simulink model "PLL_fault_experiment"  (R2025a)
settings: Solver=FixedStepAuto  StartTime=0.0  StopTime=1  FixedStep=Ts  RelTol=1e-3
values from neighbouring files (symbols this model uses):
  C_dc = 2.25    [PLLpara.m]
  Cf1 = 0.01    [PLLpara.m]
  Cf2 = 0.01    [PLLpara.m]
  dt_sag = t_c    [GFMPara.m]    (also in GFMPara_exp.m; PLLpara.m; VFMPara.m; VFMPara_exp.m)
  f_switching = 20e3    (= 20000)    [GFMPara_exp.m]    (also in PLLpara.m = 10000; VFMPara_exp.m)
  Id0 = Id    [PLLpara.m]
  Iq01 = 0    [PLLpara.m]
  Iq02 = (Ug*cos(asin((Xg*Id+Rg*Iq)/Ug))+Id*Rg-Iq*Xg)*Cf2+Iq    [PLLpara.m]
  ki_pll1 = ki    [PLLpara.m]
  kp_pll1 = kp    [PLLpara.m]
  Lc = 1e-9    (= 1e-09)    [GFMPara.m]    (also in GFMPara_exp.m; PLLpara.m; VFMPara.m; VFMPara_exp.m)
  Lf = 0.0592    [GFMPara.m]    (also in GFMPara_exp.m; PLLpara.m = 0.05; VFMPara.m = 0.05; VFMPara_exp.m = 0.05)
  Lg1 = X1    [PLLpara.m]    (also in VFMPara.m; VFMPara_exp.m)
  Lgg = Xgg    [PLLpara.m]    (also in VFMPara.m; VFMPara_exp.m)
  Rf = 1e-3    (= 0.001)    [PLLpara.m]
  Rg1 = R1    [PLLpara.m]    (also in VFMPara.m; VFMPara_exp.m = 4*R1/5)
  Rgg = Rgg    [PLLpara.m]    (also in VFMPara.m; VFMPara_exp.m)
  Sbase = 1    [GFMPara.m]    (also in GFMPara_exp.m; PLLpara.m; VFMPara.m; VFMPara_exp.m)
  t0 = t_sim_start +t_start    [PLLpara.m]    (also in VFMPara_exp.m)
  t0_sag = t_sim_start +t_start    [GFMPara.m]    (also in GFMPara_exp.m; PLLpara.m = 20; VFMPara.m; VFMPara_exp.m = 20)
  Tc = 1/f_switching    (= 5e-05)    [GFMPara_exp.m]    (also in PLLpara.m = 0.0001; VFMPara_exp.m)
  tc = t_c    [PLLpara.m]    (also in VFMPara_exp.m)
  Ts = 1/Fs    (= 1e-05)    [GFMPara.m]    (also in GFMPara_exp.m = 1e-06; PLLpara.m = 1e-06; VFMPara.m = 5e-06; VFMPara_exp.m = 1e-06)
  v_sag = Ug_fault    [GFMPara.m]    (also in GFMPara_exp.m; PLLpara.m; VFMPara.m; VFMPara_exp.m)
  Vbase = 1    [GFMPara.m]    (also in GFMPara_exp.m; PLLpara.m; VFMPara.m; VFMPara_exp.m)
  Vdc = 2.5    [PLLpara.m]
  w_i_GFL1 = 1100 *2*pi    (= 6911.5038379)    [PLLpara.m]
  w_i_GFL2 = 1100 *2*pi    (= 6911.5038379)    [PLLpara.m]
  w_pll1 = 10 *2*pi    (= 62.8318530718)    [PLLpara.m]
  w_tau1 = 1500 *2*pi    (= 9424.77796077)    [PLLpara.m]
  Wbase = 2*pi*50    (= 314.159265359)    [GFMPara.m]    (also in GFMPara_exp.m; PLLpara.m; VFMPara.m; VFMPara_exp.m)
  Zbase = Vbase/Ibase    (= 1)    [GFMPara.m]    (also in GFMPara_exp.m; PLLpara.m; VFMPara.m; VFMPara_exp.m)
undefined symbols (not defined in the file or in its folder): DiscIntNeverNeededParam, initial, position, postfault_SEP, sigbuilder_block, w_max, w_min, Ws
libraries: spsVoltageMeasurementLib x80, spsCurrentMeasurementLib x75, spsIdealSwitchLib x30, spsThreePhaseSeriesRLCBranchLib x21, spsControlledVoltageSourceLib x18, spsSeriesRLCBranchLib x11, powerlib_extras x10, spsHalfBridgeConverterLib x6, spsThreePhaseBreakerLib x6, spsDCVoltageSourceLib x4, spsThreePhaseFaultLib x3, cstblocks x2
(part 3 of 5)

== system PLL_fault_experiment/measurement12 ==
  Mux1 : Mux  Inputs=3
  Mux2 : Mux  Inputs=3
  ila : spsCurrentMeasurementLib/Current Measurement  PhasorSimulation=off  OutputType=Complex  PSBequivalent=0
  ilb : spsCurrentMeasurementLib/Current Measurement  PhasorSimulation=off  OutputType=Complex  PSBequivalent=0
  ilc : spsCurrentMeasurementLib/Current Measurement  PhasorSimulation=off  OutputType=Complex  PSBequivalent=0
  vca measure : spsVoltageMeasurementLib/Voltage Measurement  PhasorSimulation=off  OutputType=Complex  PSBequivalent=0
  vcb measure : spsVoltageMeasurementLib/Voltage Measurement  PhasorSimulation=off  OutputType=Complex  PSBequivalent=0
  vcc measure : spsVoltageMeasurementLib/Voltage Measurement  PhasorSimulation=off  OutputType=Complex  PSBequivalent=0
  a : PMIOPort  Side=Left
  b : PMIOPort  Port=2  Side=Left
  c : PMIOPort  Port=3  Side=Left
  n : PMIOPort  Port=4  Side=Left
  A : PMIOPort  Port=5  Side=Right
  B : PMIOPort  Port=6  Side=Right
  C : PMIOPort  Port=7  Side=Right
  N : PMIOPort  Port=8  Side=Right
  Iabc : Outport
  Vabc : Outport  Port=2
  wires:
  ila/1 -> Mux2/1
  ilb/1 -> Mux2/2
  ilc/1 -> Mux2/3
  Mux2/1 -> Iabc/1
  vcb measure/1 -> Mux1/2
  vca measure/1 -> Mux1/1
  vcc measure/1 -> Mux1/3
  Mux1/1 -> Vabc/1
  connections:
  a/RConn1 -- ila/LConn1
  ila/RConn1 -- A/RConn1 -- vca measure/LConn1
  ilb/LConn1 -- b/RConn1
  ilb/RConn1 -- B/RConn1 -- vcb measure/LConn1
  c/RConn1 -- ilc/LConn1
  C/RConn1 -- ilc/RConn1 -- vcc measure/LConn1
  n/RConn1 -- vcc measure/LConn2 -- vcb measure/LConn2 -- vca measure/LConn2 -- N/RConn1

== system PLL_fault_experiment/measurement13 ==
  Mux1 : Mux  Inputs=3
  Mux2 : Mux  Inputs=3
  ila : spsCurrentMeasurementLib/Current Measurement  PhasorSimulation=off  OutputType=Complex  PSBequivalent=0
  ilb : spsCurrentMeasurementLib/Current Measurement  PhasorSimulation=off  OutputType=Complex  PSBequivalent=0
  ilc : spsCurrentMeasurementLib/Current Measurement  PhasorSimulation=off  OutputType=Complex  PSBequivalent=0
  vca measure : spsVoltageMeasurementLib/Voltage Measurement  PhasorSimulation=off  OutputType=Complex  PSBequivalent=0
  vcb measure : spsVoltageMeasurementLib/Voltage Measurement  PhasorSimulation=off  OutputType=Complex  PSBequivalent=0
  vcc measure : spsVoltageMeasurementLib/Voltage Measurement  PhasorSimulation=off  OutputType=Complex  PSBequivalent=0
  a : PMIOPort  Side=Left
  b : PMIOPort  Port=2  Side=Left
  c : PMIOPort  Port=3  Side=Left
  n : PMIOPort  Port=4  Side=Left
  A : PMIOPort  Port=5  Side=Right
  B : PMIOPort  Port=6  Side=Right
  C : PMIOPort  Port=7  Side=Right
  N : PMIOPort  Port=8  Side=Right
  Iabc : Outport
  Vabc : Outport  Port=2
  wires:
  ila/1 -> Mux2/1
  ilb/1 -> Mux2/2
  ilc/1 -> Mux2/3
  Mux2/1 -> Iabc/1
  vcb measure/1 -> Mux1/2
  vca measure/1 -> Mux1/1
  vcc measure/1 -> Mux1/3
  Mux1/1 -> Vabc/1
  connections:
  a/RConn1 -- ila/LConn1
  ila/RConn1 -- A/RConn1 -- vca measure/LConn1
  ilb/LConn1 -- b/RConn1
  ilb/RConn1 -- B/RConn1 -- vcb measure/LConn1
  c/RConn1 -- ilc/LConn1
  C/RConn1 -- ilc/RConn1 -- vcc measure/LConn1
  n/RConn1 -- vcc measure/LConn2 -- vcb measure/LConn2 -- vca measure/LConn2 -- N/RConn1

== system PLL_fault_experiment/measurement14 ==
  Mux1 : Mux  Inputs=3
  Mux2 : Mux  Inputs=3
  ila : spsCurrentMeasurementLib/Current Measurement  PhasorSimulation=off  OutputType=Complex  PSBequivalent=0
  ilb : spsCurrentMeasurementLib/Current Measurement  PhasorSimulation=off  OutputType=Complex  PSBequivalent=0
  ilc : spsCurrentMeasurementLib/Current Measurement  PhasorSimulation=off  OutputType=Complex  PSBequivalent=0
  vca measure : spsVoltageMeasurementLib/Voltage Measurement  PhasorSimulation=off  OutputType=Complex  PSBequivalent=0
  vcb measure : spsVoltageMeasurementLib/Voltage Measurement  PhasorSimulation=off  OutputType=Complex  PSBequivalent=0
  vcc measure : spsVoltageMeasurementLib/Voltage Measurement  PhasorSimulation=off  OutputType=Complex  PSBequivalent=0
  a : PMIOPort  Side=Left
  b : PMIOPort  Port=2  Side=Left
  c : PMIOPort  Port=3  Side=Left
  n : PMIOPort  Port=4  Side=Left
  A : PMIOPort  Port=5  Side=Right
  B : PMIOPort  Port=6  Side=Right
  C : PMIOPort  Port=7  Side=Right
  N : PMIOPort  Port=8  Side=Right
  Iabc : Outport
  Vabc : Outport  Port=2
  wires:
  ila/1 -> Mux2/1
  ilb/1 -> Mux2/2
  ilc/1 -> Mux2/3
  Mux2/1 -> Iabc/1
  vcb measure/1 -> Mux1/2
  vca measure/1 -> Mux1/1
  vcc measure/1 -> Mux1/3
  Mux1/1 -> Vabc/1
  connections:
  a/RConn1 -- ila/LConn1
  ila/RConn1 -- A/RConn1 -- vca measure/LConn1
  ilb/LConn1 -- b/RConn1
  ilb/RConn1 -- B/RConn1 -- vcb measure/LConn1
  c/RConn1 -- ilc/LConn1
  C/RConn1 -- ilc/RConn1 -- vcc measure/LConn1
  n/RConn1 -- vcc measure/LConn2 -- vcb measure/LConn2 -- vca measure/LConn2 -- N/RConn1

== system PLL_fault_experiment/measurement15 ==
  Mux1 : Mux  Inputs=3
  Mux2 : Mux  Inputs=3
  ila : spsCurrentMeasurementLib/Current Measurement  PhasorSimulation=off  OutputType=Complex  PSBequivalent=0
  ilb : spsCurrentMeasurementLib/Current Measurement  PhasorSimulation=off  OutputType=Complex  PSBequivalent=0
  ilc : spsCurrentMeasurementLib/Current Measurement  PhasorSimulation=off  OutputType=Complex  PSBequivalent=0
  vca measure : spsVoltageMeasurementLib/Voltage Measurement  PhasorSimulation=off  OutputType=Complex  PSBequivalent=0
  vcb measure : spsVoltageMeasurementLib/Voltage Measurement  PhasorSimulation=off  OutputType=Complex  PSBequivalent=0
  vcc measure : spsVoltageMeasurementLib/Voltage Measurement  PhasorSimulation=off  OutputType=Complex  PSBequivalent=0
  a : PMIOPort  Side=Left
  b : PMIOPort  Port=2  Side=Left
  c : PMIOPort  Port=3  Side=Left
  n : PMIOPort  Port=4  Side=Left
  A : PMIOPort  Port=5  Side=Right
  B : PMIOPort  Port=6  Side=Right
  C : PMIOPort  Port=7  Side=Right
  N : PMIOPort  Port=8  Side=Right
  Iabc : Outport
  Vabc : Outport  Port=2
  wires:
  ila/1 -> Mux2/1
  ilb/1 -> Mux2/2
  ilc/1 -> Mux2/3
  Mux2/1 -> Iabc/1
  vcb measure/1 -> Mux1/2
  vca measure/1 -> Mux1/1
  vcc measure/1 -> Mux1/3
  Mux1/1 -> Vabc/1
  connections:
  a/RConn1 -- ila/LConn1
  ila/RConn1 -- A/RConn1 -- vca measure/LConn1
  ilb/LConn1 -- b/RConn1
  ilb/RConn1 -- B/RConn1 -- vcb measure/LConn1
  c/RConn1 -- ilc/LConn1
  C/RConn1 -- ilc/RConn1 -- vcc measure/LConn1
  n/RConn1 -- vcc measure/LConn2 -- vcb measure/LConn2 -- vca measure/LConn2 -- N/RConn1

== system PLL_fault_experiment/measurement2 ==
  Mux1 : Mux  Inputs=3
  Mux2 : Mux  Inputs=3
  ila : spsCurrentMeasurementLib/Current Measurement  PhasorSimulation=off  OutputType=Complex  PSBequivalent=0
  ilb : spsCurrentMeasurementLib/Current Measurement  PhasorSimulation=off  OutputType=Complex  PSBequivalent=0
  ilc : spsCurrentMeasurementLib/Current Measurement  PhasorSimulation=off  OutputType=Complex  PSBequivalent=0
  vca measure : spsVoltageMeasurementLib/Voltage Measurement  PhasorSimulation=off  OutputType=Complex  PSBequivalent=0
  vcb measure : spsVoltageMeasurementLib/Voltage Measurement  PhasorSimulation=off  OutputType=Complex  PSBequivalent=0
  vcc measure : spsVoltageMeasurementLib/Voltage Measurement  PhasorSimulation=off  OutputType=Complex  PSBequivalent=0
  a : PMIOPort  Side=Left
  b : PMIOPort  Port=2  Side=Left
  c : PMIOPort  Port=3  Side=Left
  n : PMIOPort  Port=4  Side=Left
  A : PMIOPort  Port=5  Side=Right
  B : PMIOPort  Port=6  Side=Right
  C : PMIOPort  Port=7  Side=Right
  N : PMIOPort  Port=8  Side=Right
  Iabc : Outport
  Vabc : Outport  Port=2
  wires:
  ila/1 -> Mux2/1
  ilb/1 -> Mux2/2
  ilc/1 -> Mux2/3
  Mux2/1 -> Iabc/1
  vcb measure/1 -> Mux1/2
  vca measure/1 -> Mux1/1
  vcc measure/1 -> Mux1/3
  Mux1/1 -> Vabc/1
  connections:
  a/RConn1 -- ila/LConn1
  ila/RConn1 -- A/RConn1 -- vca measure/LConn1
  ilb/LConn1 -- b/RConn1
  ilb/RConn1 -- B/RConn1 -- vcb measure/LConn1
  c/RConn1 -- ilc/LConn1
  C/RConn1 -- ilc/RConn1 -- vcc measure/LConn1
  n/RConn1 -- vcc measure/LConn2 -- vcb measure/LConn2 -- vca measure/LConn2 -- N/RConn1

== system PLL_fault_experiment/measurement3 ==
  Mux1 : Mux  Inputs=3
  Mux2 : Mux  Inputs=3
  ila : spsCurrentMeasurementLib/Current Measurement  PhasorSimulation=off  OutputType=Complex  PSBequivalent=0
  ilb : spsCurrentMeasurementLib/Current Measurement  PhasorSimulation=off  OutputType=Complex  PSBequivalent=0
  ilc : spsCurrentMeasurementLib/Current Measurement  PhasorSimulation=off  OutputType=Complex  PSBequivalent=0
  vca measure : spsVoltageMeasurementLib/Voltage Measurement  PhasorSimulation=off  OutputType=Complex  PSBequivalent=0
  vcb measure : spsVoltageMeasurementLib/Voltage Measurement  PhasorSimulation=off  OutputType=Complex  PSBequivalent=0
  vcc measure : spsVoltageMeasurementLib/Voltage Measurement  PhasorSimulation=off  OutputType=Complex  PSBequivalent=0
  a : PMIOPort  Side=Left
  b : PMIOPort  Port=2  Side=Left
  c : PMIOPort  Port=3  Side=Left
  n : PMIOPort  Port=4  Side=Left
  A : PMIOPort  Port=5  Side=Right
  B : PMIOPort  Port=6  Side=Right
  C : PMIOPort  Port=7  Side=Right
  N : PMIOPort  Port=8  Side=Right
  Iabc : Outport
  Vabc : Outport  Port=2
  wires:
  ila/1 -> Mux2/1
  ilb/1 -> Mux2/2
  ilc/1 -> Mux2/3
  Mux2/1 -> Iabc/1
  vcb measure/1 -> Mux1/2
  vca measure/1 -> Mux1/1
  vcc measure/1 -> Mux1/3
  Mux1/1 -> Vabc/1
  connections:
  a/RConn1 -- ila/LConn1
  ila/RConn1 -- A/RConn1 -- vca measure/LConn1
  ilb/LConn1 -- b/RConn1
  ilb/RConn1 -- B/RConn1 -- vcb measure/LConn1
  c/RConn1 -- ilc/LConn1
  C/RConn1 -- ilc/RConn1 -- vcc measure/LConn1
  n/RConn1 -- vcc measure/LConn2 -- vcb measure/LConn2 -- vca measure/LConn2 -- N/RConn1

== system PLL_fault_experiment/measurement4 ==
  Mux1 : Mux  Inputs=3
  Mux2 : Mux  Inputs=3
  ila : spsCurrentMeasurementLib/Current Measurement  PhasorSimulation=off  OutputType=Complex  PSBequivalent=0
  ilb : spsCurrentMeasurementLib/Current Measurement  PhasorSimulation=off  OutputType=Complex  PSBequivalent=0
  ilc : spsCurrentMeasurementLib/Current Measurement  PhasorSimulation=off  OutputType=Complex  PSBequivalent=0
  vca measure : spsVoltageMeasurementLib/Voltage Measurement  PhasorSimulation=off  OutputType=Complex  PSBequivalent=0
  vcb measure : spsVoltageMeasurementLib/Voltage Measurement  PhasorSimulation=off  OutputType=Complex  PSBequivalent=0
  vcc measure : spsVoltageMeasurementLib/Voltage Measurement  PhasorSimulation=off  OutputType=Complex  PSBequivalent=0
  a : PMIOPort  Side=Left
  b : PMIOPort  Port=2  Side=Left
  c : PMIOPort  Port=3  Side=Left
  n : PMIOPort  Port=4  Side=Left
  A : PMIOPort  Port=5  Side=Right
  B : PMIOPort  Port=6  Side=Right
  C : PMIOPort  Port=7  Side=Right
  N : PMIOPort  Port=8  Side=Right
  Iabc : Outport
  Vabc : Outport  Port=2
  wires:
  ila/1 -> Mux2/1
  ilb/1 -> Mux2/2
  ilc/1 -> Mux2/3
  Mux2/1 -> Iabc/1
  vcb measure/1 -> Mux1/2
  vca measure/1 -> Mux1/1
  vcc measure/1 -> Mux1/3
  Mux1/1 -> Vabc/1
  connections:
  a/RConn1 -- ila/LConn1
  ila/RConn1 -- A/RConn1 -- vca measure/LConn1
  ilb/LConn1 -- b/RConn1
  ilb/RConn1 -- B/RConn1 -- vcb measure/LConn1
  c/RConn1 -- ilc/LConn1
  C/RConn1 -- ilc/RConn1 -- vcc measure/LConn1
  n/RConn1 -- vcc measure/LConn2 -- vcb measure/LConn2 -- vca measure/LConn2 -- N/RConn1

== system PLL_fault_experiment/measurement5 ==
  Mux1 : Mux  Inputs=3
  Mux2 : Mux  Inputs=3
  ila : spsCurrentMeasurementLib/Current Measurement  PhasorSimulation=off  OutputType=Complex  PSBequivalent=0
  ilb : spsCurrentMeasurementLib/Current Measurement  PhasorSimulation=off  OutputType=Complex  PSBequivalent=0
  ilc : spsCurrentMeasurementLib/Current Measurement  PhasorSimulation=off  OutputType=Complex  PSBequivalent=0
  vca measure : spsVoltageMeasurementLib/Voltage Measurement  PhasorSimulation=off  OutputType=Complex  PSBequivalent=0
  vcb measure : spsVoltageMeasurementLib/Voltage Measurement  PhasorSimulation=off  OutputType=Complex  PSBequivalent=0
  vcc measure : spsVoltageMeasurementLib/Voltage Measurement  PhasorSimulation=off  OutputType=Complex  PSBequivalent=0
  a : PMIOPort  Side=Left
  b : PMIOPort  Port=2  Side=Left
  c : PMIOPort  Port=3  Side=Left
  n : PMIOPort  Port=4  Side=Left
  A : PMIOPort  Port=5  Side=Right
  B : PMIOPort  Port=6  Side=Right
  C : PMIOPort  Port=7  Side=Right
  N : PMIOPort  Port=8  Side=Right
  Iabc : Outport
  Vabc : Outport  Port=2
  wires:
  ila/1 -> Mux2/1
  ilb/1 -> Mux2/2
  ilc/1 -> Mux2/3
  Mux2/1 -> Iabc/1
  vcb measure/1 -> Mux1/2
  vca measure/1 -> Mux1/1
  vcc measure/1 -> Mux1/3
  Mux1/1 -> Vabc/1
  connections:
  a/RConn1 -- ila/LConn1
  ila/RConn1 -- A/RConn1 -- vca measure/LConn1
  ilb/LConn1 -- b/RConn1
  ilb/RConn1 -- B/RConn1 -- vcb measure/LConn1
  c/RConn1 -- ilc/LConn1
  C/RConn1 -- ilc/RConn1 -- vcc measure/LConn1
  n/RConn1 -- vcc measure/LConn2 -- vcb measure/LConn2 -- vca measure/LConn2 -- N/RConn1

== system PLL_fault_experiment/measurement6 ==
  Mux1 : Mux  Inputs=3
  Mux2 : Mux  Inputs=3
  ila : spsCurrentMeasurementLib/Current Measurement  PhasorSimulation=off  OutputType=Complex  PSBequivalent=0
  ilb : spsCurrentMeasurementLib/Current Measurement  PhasorSimulation=off  OutputType=Complex  PSBequivalent=0
  ilc : spsCurrentMeasurementLib/Current Measurement  PhasorSimulation=off  OutputType=Complex  PSBequivalent=0
  vca measure : spsVoltageMeasurementLib/Voltage Measurement  PhasorSimulation=off  OutputType=Complex  PSBequivalent=0
  vcb measure : spsVoltageMeasurementLib/Voltage Measurement  PhasorSimulation=off  OutputType=Complex  PSBequivalent=0
  vcc measure : spsVoltageMeasurementLib/Voltage Measurement  PhasorSimulation=off  OutputType=Complex  PSBequivalent=0
  a : PMIOPort  Side=Left
  b : PMIOPort  Port=2  Side=Left
  c : PMIOPort  Port=3  Side=Left
  n : PMIOPort  Port=4  Side=Left
  A : PMIOPort  Port=5  Side=Right
  B : PMIOPort  Port=6  Side=Right
  C : PMIOPort  Port=7  Side=Right
  N : PMIOPort  Port=8  Side=Right
  Iabc : Outport
  Vabc : Outport  Port=2
  wires:
  ila/1 -> Mux2/1
  ilb/1 -> Mux2/2
  ilc/1 -> Mux2/3
  Mux2/1 -> Iabc/1
  vcb measure/1 -> Mux1/2
  vca measure/1 -> Mux1/1
  vcc measure/1 -> Mux1/3
  Mux1/1 -> Vabc/1
  connections:
  a/RConn1 -- ila/LConn1
  ila/RConn1 -- A/RConn1 -- vca measure/LConn1
  ilb/LConn1 -- b/RConn1
  ilb/RConn1 -- B/RConn1 -- vcb measure/LConn1
  c/RConn1 -- ilc/LConn1
  C/RConn1 -- ilc/RConn1 -- vcc measure/LConn1
  n/RConn1 -- vcc measure/LConn2 -- vcb measure/LConn2 -- vca measure/LConn2 -- N/RConn1

== system PLL_fault_experiment/measurement7 ==
  Mux1 : Mux  Inputs=3
  Mux2 : Mux  Inputs=3
  ila : spsCurrentMeasurementLib/Current Measurement  PhasorSimulation=off  OutputType=Complex  PSBequivalent=0
  ilb : spsCurrentMeasurementLib/Current Measurement  PhasorSimulation=off  OutputType=Complex  PSBequivalent=0
  ilc : spsCurrentMeasurementLib/Current Measurement  PhasorSimulation=off  OutputType=Complex  PSBequivalent=0
  vca measure : spsVoltageMeasurementLib/Voltage Measurement  PhasorSimulation=off  OutputType=Complex  PSBequivalent=0
  vcb measure : spsVoltageMeasurementLib/Voltage Measurement  PhasorSimulation=off  OutputType=Complex  PSBequivalent=0
  vcc measure : spsVoltageMeasurementLib/Voltage Measurement  PhasorSimulation=off  OutputType=Complex  PSBequivalent=0
  a : PMIOPort  Side=Left
  b : PMIOPort  Port=2  Side=Left
  c : PMIOPort  Port=3  Side=Left
  n : PMIOPort  Port=4  Side=Left
  A : PMIOPort  Port=5  Side=Right
  B : PMIOPort  Port=6  Side=Right
  C : PMIOPort  Port=7  Side=Right
  N : PMIOPort  Port=8  Side=Right
  Iabc : Outport
  Vabc : Outport  Port=2
  wires:
  ila/1 -> Mux2/1
  ilb/1 -> Mux2/2
  ilc/1 -> Mux2/3
  Mux2/1 -> Iabc/1
  vcb measure/1 -> Mux1/2
  vca measure/1 -> Mux1/1
  vcc measure/1 -> Mux1/3
  Mux1/1 -> Vabc/1
  connections:
  a/RConn1 -- ila/LConn1
  ila/RConn1 -- A/RConn1 -- vca measure/LConn1
  ilb/LConn1 -- b/RConn1
  ilb/RConn1 -- B/RConn1 -- vcb measure/LConn1
  c/RConn1 -- ilc/LConn1
  C/RConn1 -- ilc/RConn1 -- vcc measure/LConn1
  n/RConn1 -- vcc measure/LConn2 -- vcb measure/LConn2 -- vca measure/LConn2 -- N/RConn1

== system PLL_fault_experiment/measurement8 ==
  Mux1 : Mux  Inputs=3
  Mux2 : Mux  Inputs=3
  ila : spsCurrentMeasurementLib/Current Measurement  PhasorSimulation=off  OutputType=Complex  PSBequivalent=0
  ilb : spsCurrentMeasurementLib/Current Measurement  PhasorSimulation=off  OutputType=Complex  PSBequivalent=0
  ilc : spsCurrentMeasurementLib/Current Measurement  PhasorSimulation=off  OutputType=Complex  PSBequivalent=0
  vca measure : spsVoltageMeasurementLib/Voltage Measurement  PhasorSimulation=off  OutputType=Complex  PSBequivalent=0
  vcb measure : spsVoltageMeasurementLib/Voltage Measurement  PhasorSimulation=off  OutputType=Complex  PSBequivalent=0
  vcc measure : spsVoltageMeasurementLib/Voltage Measurement  PhasorSimulation=off  OutputType=Complex  PSBequivalent=0
  a : PMIOPort  Side=Left
  b : PMIOPort  Port=2  Side=Left
  c : PMIOPort  Port=3  Side=Left
  n : PMIOPort  Port=4  Side=Left
  A : PMIOPort  Port=5  Side=Right
  B : PMIOPort  Port=6  Side=Right
  C : PMIOPort  Port=7  Side=Right
  N : PMIOPort  Port=8  Side=Right
  Iabc : Outport
  Vabc : Outport  Port=2
  wires:
  ila/1 -> Mux2/1
  ilb/1 -> Mux2/2
  ilc/1 -> Mux2/3
  Mux2/1 -> Iabc/1
  vcb measure/1 -> Mux1/2
  vca measure/1 -> Mux1/1
  vcc measure/1 -> Mux1/3
  Mux1/1 -> Vabc/1
  connections:
  a/RConn1 -- ila/LConn1
  ila/RConn1 -- A/RConn1 -- vca measure/LConn1
  ilb/LConn1 -- b/RConn1
  ilb/RConn1 -- B/RConn1 -- vcb measure/LConn1
  c/RConn1 -- ilc/LConn1
  C/RConn1 -- ilc/RConn1 -- vcc measure/LConn1
  n/RConn1 -- vcc measure/LConn2 -- vcb measure/LConn2 -- vca measure/LConn2 -- N/RConn1

== system PLL_fault_experiment/measurement9 ==
  Mux1 : Mux  Inputs=3
  Mux2 : Mux  Inputs=3
  ila : spsCurrentMeasurementLib/Current Measurement  PhasorSimulation=off  OutputType=Complex  PSBequivalent=0
  ilb : spsCurrentMeasurementLib/Current Measurement  PhasorSimulation=off  OutputType=Complex  PSBequivalent=0
  ilc : spsCurrentMeasurementLib/Current Measurement  PhasorSimulation=off  OutputType=Complex  PSBequivalent=0
  vca measure : spsVoltageMeasurementLib/Voltage Measurement  PhasorSimulation=off  OutputType=Complex  PSBequivalent=0
  vcb measure : spsVoltageMeasurementLib/Voltage Measurement  PhasorSimulation=off  OutputType=Complex  PSBequivalent=0
  vcc measure : spsVoltageMeasurementLib/Voltage Measurement  PhasorSimulation=off  OutputType=Complex  PSBequivalent=0
  a : PMIOPort  Side=Left
  b : PMIOPort  Port=2  Side=Left
  c : PMIOPort  Port=3  Side=Left
  n : PMIOPort  Port=4  Side=Left
  A : PMIOPort  Port=5  Side=Right
  B : PMIOPort  Port=6  Side=Right
  C : PMIOPort  Port=7  Side=Right
  N : PMIOPort  Port=8  Side=Right
  Iabc : Outport
  Vabc : Outport  Port=2
  wires:
  ila/1 -> Mux2/1
  ilb/1 -> Mux2/2
  ilc/1 -> Mux2/3
  Mux2/1 -> Iabc/1
  vcb measure/1 -> Mux1/2
  vca measure/1 -> Mux1/1
  vcc measure/1 -> Mux1/3
  Mux1/1 -> Vabc/1
  connections:
  a/RConn1 -- ila/LConn1
  ila/RConn1 -- A/RConn1 -- vca measure/LConn1
  ilb/LConn1 -- b/RConn1
  ilb/RConn1 -- B/RConn1 -- vcb measure/LConn1
  c/RConn1 -- ilc/LConn1
  C/RConn1 -- ilc/RConn1 -- vcc measure/LConn1
  n/RConn1 -- vcc measure/LConn2 -- vcb measure/LConn2 -- vca measure/LConn2 -- N/RConn1

== system PLL_fault_experiment/AC Infinite Bus (Voltage Type)1/PQ Calculation (dq-Frame)1 ==
  note: Power calculation.
      |
      | Author(s): Yitong Li
      |
      | Notes:
      |
      | The calculation is done in dq frame.
  vdq : Inport
  idq : Inport  Port=2
  Mux : Mux  Inputs=2
  Mux1 : Mux  Inputs=2
  P = vd*id+vq*iq : Fcn  Expr=u[1]*u[3]+u[2]*u[4]
  Q = -vd*iq+vq*id : Fcn  Expr=-u[1]*u[4]+u[2]*u[3]
  pq : Outport
  wires:
  Mux/1 -> pq/1
  P = vd*id+vq*iq/1 -> Mux/1
  vdq/1 -> Mux1/1
  idq/1 -> Mux1/2
  Mux1/1 -> P = vd*id+vq*iq/1, Q = -vd*iq+vq*id/1
  Q = -vd*iq+vq*id/1 -> Mux/2

== system PLL_fault_experiment/AC Infinite Bus (Voltage Type)1/abc -> dq (Power-Invariant)1 ==
  note: Frame transformation from abc to dq.
      |
      | Author(s): Yitong Li
      |
      | Notes:
      |
      | The transformation is power-invariant.
      |
      | theta is the angle that d axis leads a axis.
      |
      | q axis leads d axis by 90 degrees.
  abc : Inport
  theta : Inport  Port=2
  ->d : Fcn  Expr=cos(u(4))*u(1) + cos(u(4)-2/3*pi)*u(2) + cos(u(4)-4/3*pi)*u(3)
  ->q : Fcn  Expr=-sin(u(4))*u(1) - sin(u(4)-2/3*pi)*u(2) - sin(u(4)-4/3*pi)*u(3)
  Gain : Gain  Gain=sqrt(2/3)
  Mux5 : Mux  Inputs=2
  Mux6 : Mux  Inputs=2
  dq : Outport
  wires:
  abc/1 -> Gain/1
  ->d/1 -> Mux6/1
  Gain/1 -> Mux5/1
  theta/1 -> Mux5/2
  ->q/1 -> Mux6/2
  Mux6/1 -> dq/1
  Mux5/1 -> ->d/1, ->q/1

== system PLL_fault_experiment/AC Infinite Bus (Voltage Type)1/dq -> abc (Power-Invariant)1 ==
  note: Frame transformation from dq to abc.
      |
      | Author(s): Yitong Li
      |
      | Notes:
      |
      | The transformation is power-invariant.
      |
      | theta is the angle that dq axis leads alpha/beta axis, specifically, d axis leads alpha axis.
  dq : Inport
  theta : Inport  Port=2
  ->a : Fcn  Expr=cos(u(3))*u(1) - sin(u(3))*u(2)
  ->b : Fcn  Expr=cos(u(3)-2/3*pi)*u(1) - sin(u(3)-2/3*pi)*u(2)
  ->c : Fcn  Expr=cos(u(3)-4/3*pi)*u(1) - sin(u(3)-4/3*pi)*u(2)
  Gain : Gain  Gain=sqrt(2/3)
  Mux5 : Mux  Inputs=2
  Mux6 : Mux  Inputs=3
  abc : Outport
  wires:
  ->b/1 -> Mux6/2
  ->a/1 -> Mux6/1
  Gain/1 -> Mux5/1
  dq/1 -> Gain/1
  ->c/1 -> Mux6/3
  Mux6/1 -> abc/1
  Mux5/1 -> ->b/1, ->a/1, ->c/1
  theta/1 -> Mux5/2

== system PLL_fault_experiment/AC Infinite Bus (Voltage Type)2/PQ Calculation (dq-Frame)1 ==
  note: Power calculation.
      |
      | Author(s): Yitong Li
      |
      | Notes:
      |
      | The calculation is done in dq frame.
  vdq : Inport
  idq : Inport  Port=2
  Mux : Mux  Inputs=2
  Mux1 : Mux  Inputs=2
  P = vd*id+vq*iq : Fcn  Expr=u[1]*u[3]+u[2]*u[4]
  Q = -vd*iq+vq*id : Fcn  Expr=-u[1]*u[4]+u[2]*u[3]
  pq : Outport
  wires:
  Mux/1 -> pq/1
  P = vd*id+vq*iq/1 -> Mux/1
  vdq/1 -> Mux1/1
  idq/1 -> Mux1/2
  Mux1/1 -> P = vd*id+vq*iq/1, Q = -vd*iq+vq*id/1
  Q = -vd*iq+vq*id/1 -> Mux/2

== system PLL_fault_experiment/AC Infinite Bus (Voltage Type)2/abc -> dq (Power-Invariant)1 ==
  note: Frame transformation from abc to dq.
      |
      | Author(s): Yitong Li
      |
      | Notes:
      |
      | The transformation is power-invariant.
      |
      | theta is the angle that d axis leads a axis.
      |
      | q axis leads d axis by 90 degrees.
  abc : Inport
  theta : Inport  Port=2
  ->d : Fcn  Expr=cos(u(4))*u(1) + cos(u(4)-2/3*pi)*u(2) + cos(u(4)-4/3*pi)*u(3)
  ->q : Fcn  Expr=-sin(u(4))*u(1) - sin(u(4)-2/3*pi)*u(2) - sin(u(4)-4/3*pi)*u(3)
  Gain : Gain  Gain=sqrt(2/3)
  Mux5 : Mux  Inputs=2
  Mux6 : Mux  Inputs=2
  dq : Outport
  wires:
  abc/1 -> Gain/1
  ->d/1 -> Mux6/1
  Gain/1 -> Mux5/1
  theta/1 -> Mux5/2
  ->q/1 -> Mux6/2
  Mux6/1 -> dq/1
  Mux5/1 -> ->d/1, ->q/1

== system PLL_fault_experiment/AC Infinite Bus (Voltage Type)2/dq -> abc (Power-Invariant)1 ==
  note: Frame transformation from dq to abc.
      |
      | Author(s): Yitong Li
      |
      | Notes:
      |
      | The transformation is power-invariant.
      |
      | theta is the angle that dq axis leads alpha/beta axis, specifically, d axis leads alpha axis.
  dq : Inport
  theta : Inport  Port=2
  ->a : Fcn  Expr=cos(u(3))*u(1) - sin(u(3))*u(2)
  ->b : Fcn  Expr=cos(u(3)-2/3*pi)*u(1) - sin(u(3)-2/3*pi)*u(2)
  ->c : Fcn  Expr=cos(u(3)-4/3*pi)*u(1) - sin(u(3)-4/3*pi)*u(2)
  Gain : Gain  Gain=sqrt(2/3)
  Mux5 : Mux  Inputs=2
  Mux6 : Mux  Inputs=3
  abc : Outport
  wires:
  ->b/1 -> Mux6/2
  ->a/1 -> Mux6/1
  Gain/1 -> Mux5/1
  dq/1 -> Gain/1
  ->c/1 -> Mux6/3
  Mux6/1 -> abc/1
  Mux5/1 -> ->b/1, ->a/1, ->c/1
  theta/1 -> Mux5/2

== system PLL_fault_experiment/AC Infinite Bus (Voltage Type)3/PQ Calculation (dq-Frame)1 ==
  note: Power calculation.
      |
      | Author(s): Yitong Li
      |
      | Notes:
      |
      | The calculation is done in dq frame.
  vdq : Inport
  idq : Inport  Port=2
  Mux : Mux  Inputs=2
  Mux1 : Mux  Inputs=2
  P = vd*id+vq*iq : Fcn  Expr=u[1]*u[3]+u[2]*u[4]
  Q = -vd*iq+vq*id : Fcn  Expr=-u[1]*u[4]+u[2]*u[3]
  pq : Outport
  wires:
  Mux/1 -> pq/1
  P = vd*id+vq*iq/1 -> Mux/1
  vdq/1 -> Mux1/1
  idq/1 -> Mux1/2
  Mux1/1 -> P = vd*id+vq*iq/1, Q = -vd*iq+vq*id/1
  Q = -vd*iq+vq*id/1 -> Mux/2

== system PLL_fault_experiment/AC Infinite Bus (Voltage Type)3/abc -> dq (Power-Invariant)1 ==
  note: Frame transformation from abc to dq.
      |
      | Author(s): Yitong Li
      |
      | Notes:
      |
      | The transformation is power-invariant.
      |
      | theta is the angle that d axis leads a axis.
      |
      | q axis leads d axis by 90 degrees.
  abc : Inport
  theta : Inport  Port=2
  ->d : Fcn  Expr=cos(u(4))*u(1) + cos(u(4)-2/3*pi)*u(2) + cos(u(4)-4/3*pi)*u(3)
  ->q : Fcn  Expr=-sin(u(4))*u(1) - sin(u(4)-2/3*pi)*u(2) - sin(u(4)-4/3*pi)*u(3)
  Gain : Gain  Gain=sqrt(2/3)
  Mux5 : Mux  Inputs=2
  Mux6 : Mux  Inputs=2
  dq : Outport
  wires:
  abc/1 -> Gain/1
  ->d/1 -> Mux6/1
  Gain/1 -> Mux5/1
  theta/1 -> Mux5/2
  ->q/1 -> Mux6/2
  Mux6/1 -> dq/1
  Mux5/1 -> ->d/1, ->q/1

== system PLL_fault_experiment/AC Infinite Bus (Voltage Type)3/dq -> abc (Power-Invariant)1 ==
  note: Frame transformation from dq to abc.
      |
      | Author(s): Yitong Li
      |
      | Notes:
      |
      | The transformation is power-invariant.
      |
      | theta is the angle that dq axis leads alpha/beta axis, specifically, d axis leads alpha axis.
  dq : Inport
  theta : Inport  Port=2
  ->a : Fcn  Expr=cos(u(3))*u(1) - sin(u(3))*u(2)
  ->b : Fcn  Expr=cos(u(3)-2/3*pi)*u(1) - sin(u(3)-2/3*pi)*u(2)
  ->c : Fcn  Expr=cos(u(3)-4/3*pi)*u(1) - sin(u(3)-4/3*pi)*u(2)
  Gain : Gain  Gain=sqrt(2/3)
  Mux5 : Mux  Inputs=2
  Mux6 : Mux  Inputs=3
  abc : Outport
  wires:
  ->b/1 -> Mux6/2
  ->a/1 -> Mux6/1
  Gain/1 -> Mux5/1
  dq/1 -> Gain/1
  ->c/1 -> Mux6/3
  Mux6/1 -> abc/1
  Mux5/1 -> ->b/1, ->a/1, ->c/1
  theta/1 -> Mux5/2

== system PLL_fault_experiment/Grid-Following Inverter (Simulink Block)1/Anti-aliasing Filters (7)3 ==
  dq : Inport  PortDimensions=2
  2nd-Order Filter : powerlib_extras/Discrete  Control Blocks/Discrete  2nd-Order Filter  FilterType=Lowpass  Fo=Fc  Zeta=0.707  Ts=Ts  Initialize=off  Vac_Init=[0.8 -25 60]  Vdc_Init=-0.4  PlotResponse=off  param1=[1 2000 0.2]
  2nd-Order Filter1 : powerlib_extras/Discrete  Control Blocks/Discrete  2nd-Order Filter  FilterType=Lowpass  Fo=Fc  Zeta=0.707  Ts=Ts  Initialize=off  Vac_Init=[0.8 -25 60]  Vdc_Init=-0.4  PlotResponse=off  param1=[1 5000 0.1]
  Demux : Demux  Outputs=2
      settings: DisplayOption=none
  Mux : Mux  Inputs=2
  " dq*" : Outport  VectorParamsAs1DForOutWhenUnconnected=off
  wires:
  Demux/2 -> 2nd-Order Filter1/1
  2nd-Order Filter1/1 -> Mux/2
  Mux/1 -> " dq*"/1
  2nd-Order Filter/1 -> Mux/1
  dq/1 -> Demux/1
  Demux/1 -> 2nd-Order Filter/1

== system PLL_fault_experiment/Grid-Following Inverter (Simulink Block)1/Current Controller ==
  iIdq* : Inport  SampleTime=Tc
  iIdq : Inport  Port=2  SampleTime=Tc
  vdq : Inport  Port=3  SampleTime=Tc
  enable : Inport  Port=4  SampleTime=Tc
  Constant : Constant  Value=Kcd
  Demux1 : Demux  Outputs=2
  Demux2 : Demux  Outputs=2
  Demux3 : Demux  Outputs=2
  Mux : Mux  Inputs=2
  PI-DT-Estimated d : Subsystem  mask{Lf=Lf, Kg=Kg, Kp=Kp, Ki=Ki, xmax=vdmax, xmin=-vdmax, Ts=Ts}
      mask prompts: Lf "Inductance"; Kg "Estimator Gain"; Kp "Proportional Gain"; Ki "Integral Gain"; xmax "Upper Limit"; xmin "Lower Limit"; Ts "Sampling Time"
  PI-DT-Estimated q : Subsystem  mask{Lf=Lf, Kg=Kg, Kp=Kp, Ki=Ki, xmax=vqmax, xmin=-vqmax, Ts=Ts}
      mask prompts: Lf "Inductance"; Kg "Estimator Gain"; Kp "Proportional Gain"; Ki "Integral Gain"; xmax "Upper Limit"; xmin "Lower Limit"; Ts "Sampling Time"
  Product : Product  Inputs=3
  Product1 : Product  Inputs=3
  sum_d : Sum  Inputs=+-
  sum_q : Sum
  wLd : Gain  Gain=Wbase*Lf
  wLq : Gain  Gain=Wbase*Lf
  vidq* : Outport  SampleTime=Tc
  wires:
  Constant/1 -> Product1/1, Product/2
  Product1/1 -> sum_d/2
  wLq/1 -> Product1/2
  Product/1 -> sum_q/1
  wLd/1 -> Product/1
  enable/1 -> Product/3, PI-DT-Estimated d/1(enable), Product1/3, PI-DT-Estimated q/4(enable)
  Demux2/2 -> PI-DT-Estimated q/3(reference)
  Demux2/1 -> PI-DT-Estimated d/2(reference)
  iIdq*/1 -> Demux2/1
  Demux3/1 -> PI-DT-Estimated d/3(initial)
  Demux3/2 -> PI-DT-Estimated q/2(initial)
  PI-DT-Estimated q/1(Out) -> sum_q/2
  vdq/1 -> Demux3/1
  PI-DT-Estimated d/1(Out) -> sum_d/1
  Mux/1 -> vidq*/1
  Demux1/2 -> wLq/1, PI-DT-Estimated q/1(actual)
  Demux1/1 -> PI-DT-Estimated d/4(actual), wLd/1
  iIdq/1 -> Demux1/1
  sum_q/1 -> Mux/2
  sum_d/1 -> Mux/1

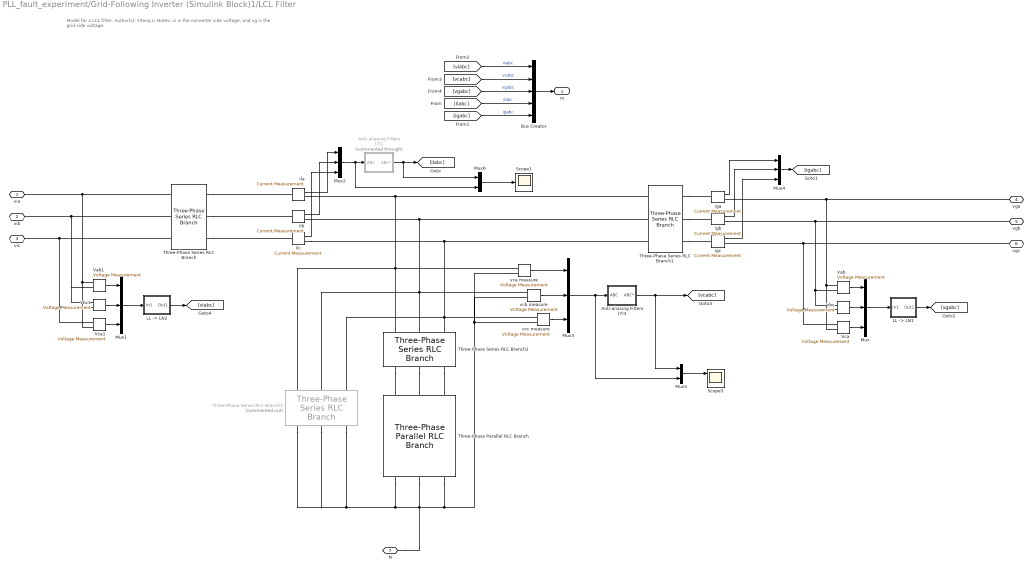
== system PLL_fault_experiment/Grid-Following Inverter (Simulink Block)1/LCL Filter ==
  note: Model for a LCL filter.
      |
      | Author(s): Yitong Li
      |
      | Notes:
      |
      | vi is the converter side voltage, and vg is the grid side voltage.
  Anti-aliasing Filters (7)1 : Subsystem  Commented=through  mask(Anti-aliasing (2nd order lowpass)){Fc=f_switching, Ts=Ts}
      mask prompts: Fc "Cut-off frequency (Hz):"; Ts "Sample time:"
  Anti-aliasing Filters (7)3 : Subsystem  mask(Anti-aliasing (2nd order lowpass)){Fc=f_switching*2, Ts=Ts}
      mask prompts: Fc "Cut-off frequency (Hz):"; Ts "Sample time:"
  Bus Creator : BusCreator  Inputs=5
  "LL -> LN1" : Subsystem  AncestorBlock=|
      | SimplusGT/Grid-Forming Inverter
      | (Simulink Block)/LCL Filter/LL -> LN1
  "LL -> LN2" : Subsystem  AncestorBlock=|
      | SimplusGT/Grid-Forming Inverter
      | (Simulink Block)/LCL Filter/LL -> LN1
  Mux{,1..4} (5 alike) : Mux  Inputs=3
  Mux5 : Mux  Inputs=2
  Mux6 : Mux  Inputs=2
  Scope1 : Scope
      settings: ActiveDisplayYMinimum=-1.56319  ActiveDisplayYMaximum=1.25944
  Scope3 : Scope  NumInputPorts=2
      settings: ActiveDisplayYMinimum=-1.53219  ActiveDisplayYMaximum=1.27746  DataLoggingVariableName=ScopeData17
  Three-Phase Parallel RLC Branch : spsThreePhaseParallelRLCBranchLib/Three-Phase Parallel RLC Branch  LConnTagsString=A|B|C  RConnTagsString=A|B|C  BranchType=RL  Resistance=2*(Vbase^2/Sbase)  Inductance=0.05*(Vbase^2/Sbase)/Wbase  Capacitance=0.01*(Vbase^2/Sbase)/Wbase  Measurements=None
  Three-Phase Series RLC Branch : spsThreePhaseSeriesRLCBranchLib/Three-Phase Series RLC Branch  LConnTagsString=A|B|C  RConnTagsString=A|B|C  BranchType=RL  Resistance=Rf  Inductance=Lf  Capacitance=1e-6  Measurements=None
  Three-Phase Series RLC Branch1 : spsThreePhaseSeriesRLCBranchLib/Three-Phase Series RLC Branch  LConnTagsString=A|B|C  RConnTagsString=A|B|C  BranchType=RL  Resistance=Rc  Inductance=Lc  Capacitance=1e-6  Measurements=None
  Three-Phase Series RLC Branch2 : spsThreePhaseSeriesRLCBranchLib/Three-Phase Series RLC Branch  LConnTagsString=A|B|C  RConnTagsString=A|B|C  BranchType=RC  Resistance=Rd  Inductance=Lc  Capacitance=Cf  Measurements=None
  Three-Phase Series RLC Branch3 : spsThreePhaseSeriesRLCBranchLib/Three-Phase Series RLC Branch  Commented=on  LConnTagsString=A|B|C  RConnTagsString=A|B|C  BranchType=C  Resistance=Rd  Inductance=Lc  Capacitance=0.01*(Sbase/Vbase^2)/Wbase/100  Measurements=None
  Vab : spsVoltageMeasurementLib/Voltage Measurement  PhasorSimulation=off  OutputType=Complex  PSBequivalent=0
  Vab1 : spsVoltageMeasurementLib/Voltage Measurement  PhasorSimulation=off  OutputType=Complex  PSBequivalent=0
  Vbc : spsVoltageMeasurementLib/Voltage Measurement  PhasorSimulation=off  OutputType=Complex  PSBequivalent=0
  Vbc1 : spsVoltageMeasurementLib/Voltage Measurement  PhasorSimulation=off  OutputType=Complex  PSBequivalent=0
  Vca : spsVoltageMeasurementLib/Voltage Measurement  PhasorSimulation=off  OutputType=Complex  PSBequivalent=0
  Vca1 : spsVoltageMeasurementLib/Voltage Measurement  PhasorSimulation=off  OutputType=Complex  PSBequivalent=0
  iga : spsCurrentMeasurementLib/Current Measurement  PhasorSimulation=off  OutputType=Complex  PSBequivalent=0
  igb : spsCurrentMeasurementLib/Current Measurement  PhasorSimulation=off  OutputType=Complex  PSBequivalent=0
  igc : spsCurrentMeasurementLib/Current Measurement  PhasorSimulation=off  OutputType=Complex  PSBequivalent=0
  ila : spsCurrentMeasurementLib/Current Measurement  PhasorSimulation=off  OutputType=Complex  PSBequivalent=0
  ilb : spsCurrentMeasurementLib/Current Measurement  PhasorSimulation=off  OutputType=Complex  PSBequivalent=0
  ilc : spsCurrentMeasurementLib/Current Measurement  PhasorSimulation=off  OutputType=Complex  PSBequivalent=0
  vca measure : spsVoltageMeasurementLib/Voltage Measurement  PhasorSimulation=off  OutputType=Complex  PSBequivalent=0
  vcb measure : spsVoltageMeasurementLib/Voltage Measurement  PhasorSimulation=off  OutputType=Complex  PSBequivalent=0
  vcc measure : spsVoltageMeasurementLib/Voltage Measurement  PhasorSimulation=off  OutputType=Complex  PSBequivalent=0
  via : PMIOPort  Side=Left
  vib : PMIOPort  Port=2  Side=Left
  vic : PMIOPort  Port=3  Side=Left
  vga : PMIOPort  Port=4  Side=Right
  vgb : PMIOPort  Port=5  Side=Right
  vgc : PMIOPort  Port=6  Side=Right
  N : PMIOPort  Port=7  Side=Left
  m : Outport
  wires:
  Mux4/1 -> [igabc]
  ilb/1 -> Mux2/2
  ila/1 -> Mux2/1
  igc/1 -> Mux4/3
  vcc measure/1 -> Mux3/3
  Vab/1 -> Mux/1
  Mux/1 -> "LL -> LN1"/1(In1)
  vca measure/1 -> Mux3/1
  vcb measure/1 -> Mux3/2
  igb/1 -> Mux4/2
  iga/1 -> Mux4/1
  Vca/1 -> Mux/3
  ilc/1 -> Mux2/3
  Vbc/1 -> Mux/2
  Bus Creator/1 -> m/1
  "LL -> LN1"/1(Out1) -> [vgabc]
  Vbc1/1 -> Mux1/2
  Vca1/1 -> Mux1/3
  Mux1/1 -> "LL -> LN2"/1(In1)
  Vab1/1 -> Mux1/1
  "LL -> LN2"/1(Out1) -> [viabc]
  [viabc] -> Bus Creator/1  "viabc"
  [vcabc] -> Bus Creator/2  "vcabc"
  [vgabc] -> Bus Creator/3  "vgabc"
  [ilabc] -> Bus Creator/4  "ilabc"
  [igabc] -> Bus Creator/5  "igabc"
  Mux3/1 -> Mux5/2, Anti-aliasing Filters (7)3/1(ABC)
  Anti-aliasing Filters (7)3/1(" ABC*") -> Mux5/1, [vcabc]
  Mux5/1 -> Scope3/1
  Mux6/1 -> Scope1/1
  Anti-aliasing Filters (7)1/1(" ABC*") -> Mux6/1, [ilabc]
  Mux2/1 -> Mux6/2, Anti-aliasing Filters (7)1/1(ABC)
  connections:
  Three-Phase Parallel RLC Branch/RConn1 -- Three-Phase Series RLC Branch3/RConn1 -- Three-Phase Series RLC Branch3/RConn2 -- Three-Phase Series RLC Branch3/RConn3 -- N/RConn1 -- Three-Phase Parallel RLC Branch/RConn2 -- Three-Phase Parallel RLC Branch/RConn3 -- vcc measure/LConn2 -- vca measure/LConn2 -- vcb measure/LConn2
  Vca/LConn1 -- Vbc/LConn2 -- igc/RConn1 -- vgc/RConn1
  Vca1/LConn1 -- Vbc1/LConn2 -- Three-Phase Series RLC Branch/LConn3 -- vic/RConn1
  Vbc1/LConn1 -- Vab1/LConn2 -- vib/RConn1 -- Three-Phase Series RLC Branch/LConn2
  Vab1/LConn1 -- Vca1/LConn2 -- Three-Phase Series RLC Branch/LConn1 -- via/RConn1
  Three-Phase Series RLC Branch1/LConn3 -- ilc/RConn1 -- Three-Phase Series RLC Branch3/LConn3 -- Three-Phase Series RLC Branch2/LConn3 -- vcc measure/LConn1
  Three-Phase Series RLC Branch1/RConn2 -- igb/LConn1
  Vbc/LConn1 -- Vab/LConn2 -- igb/RConn1 -- vgb/RConn1
  ilb/RConn1 -- Three-Phase Series RLC Branch1/LConn2 -- Three-Phase Series RLC Branch3/LConn2 -- vcb measure/LConn1 -- Three-Phase Series RLC Branch2/LConn2
  ila/RConn1 -- Three-Phase Series RLC Branch1/LConn1 -- Three-Phase Series RLC Branch3/LConn1 -- vca measure/LConn1 -- Three-Phase Series RLC Branch2/LConn1
  Vab/LConn1 -- Vca/LConn2 -- iga/RConn1 -- vga/RConn1
  Three-Phase Series RLC Branch1/RConn1 -- iga/LConn1
  Three-Phase Series RLC Branch1/RConn3 -- igc/LConn1
  Three-Phase Series RLC Branch/RConn1 -- ila/LConn1
  Three-Phase Series RLC Branch/RConn2 -- ilb/LConn1
  Three-Phase Series RLC Branch/RConn3 -- ilc/LConn1
  Three-Phase Series RLC Branch2/RConn3 -- Three-Phase Parallel RLC Branch/LConn3
  Three-Phase Series RLC Branch2/RConn2 -- Three-Phase Parallel RLC Branch/LConn2
  Three-Phase Series RLC Branch2/RConn1 -- Three-Phase Parallel RLC Branch/LConn1

== system PLL_fault_experiment/Grid-Following Inverter (Simulink Block)1/PLL (vabc -> vq) ==
  note: Measurement
  note: Gpll
  note: Phase lock loop (PLL)
      |
      | Author(s): Yitong Li
      |
      | Notes:
      |
      | vq is fed into the PI controller of the PLL.
  vabc : Inport  PortDimensions=3  SampleTime=Tc
  Constant1 : Constant
  Constant3 : Constant
  Constant4 : Constant  Value=2*pi
  Constant6 : Constant  Value=0
  Demux1 : Demux  Outputs=2
  Discrete PI : Subsystem  AncestorBlock=SimplusGT/Discrete PI  mask{Kp=kp, Ki=ki, xmax=w_max, xmin=w_min, Ts=Tc}
      mask prompts: Kp "Proportional Gain"; Ki "Integral Gain"; xmax "Upper Limit"; xmin "Lower Limit"; Ts "Sampling Time"
  Discrete-Time Integrator : DiscreteIntegrator  SampleTime=Tc  ICPrevOutput=DiscIntNeverNeededParam  ICPrevScaledInput=DiscIntNeverNeededParam
  Filter p : DiscreteTransferFcn  Numerator=[w_tau*Tc 0]  Denominator=[1+(w_tau*Tc) -1]  SampleTime=Tc
  Filter p2 : DiscreteTransferFcn  Numerator=[w_tau*Tc 0] %w_tau*Tc  Denominator="[1+(w_tau*Tc) -1]     %[1 ((w_tau*Tc)-1)]"  SampleTime=Tc
  Gain1 : Gain  Gain=Wbase
  Gain4 : Gain  Gain=1/Wbase
  Gain5 : Gain  Gain=1/pi
  Math Function1 : Math  Operator=mod  SignedPower=on
  Mux : Mux  Inputs=2
  Saturation : Saturate  UpperLimit=w_max  LowerLimit=w_min
  Scope : Scope  NumInputPorts=4
      settings: ActiveDisplayYMinimum=0.97079  ActiveDisplayYMaximum=1.02315  DataLoggingVariableName=ScopeData3
  Scope1 : Scope  NumInputPorts=4
      settings: ActiveDisplayYMinimum=-2.53693  ActiveDisplayYMaximum=2.31988  DataLoggingVariableName=ScopeData7
  Sum : Sum
  "abc -> dq (Power-Invariant)" : Subsystem  AncestorBlock=|
      | SimplusGT/abc -> dq
      | (Power-Invariant)
  w : Outport  SampleTime=Tc
  theta : Outport  Port=2  PortDimensions=1  SampleTime=Tc
  vdq : Outport  Port=3
  wires:
  vabc/1 -> "abc -> dq (Power-Invariant)"/1(abc)
  "abc -> dq (Power-Invariant)"/1(dq) -> vdq/1, Demux1/1
  Constant4/1 -> Math Function1/2
  Demux1/2 -> Filter p/1, Scope1/1, [vq]
  Constant6/1 -> Discrete PI/4(actual), Discrete PI/3(initial)
  Constant1/1 -> Discrete PI/1(enable)
  Discrete PI/1(Out) -> Scope1/4, Saturation/1
  Sum/1 -> [w], w/1, Discrete-Time Integrator/1
  Gain1/1 -> Sum/2
  [vq] -> Scope/2  "vq"
  Mux/1 -> Gain5/1
  Gain4/1 -> Scope/3
  [w] -> Gain4/1  "w"
  [theta0] -> Mux/1  "theta0"
  [vd] -> Scope/1  "vd"
  Gain5/1 -> Scope/4
  [theta] -> Mux/2  "theta"
  Demux1/1 -> [vd]
  Constant3/1 -> Gain1/1
  Math Function1/1 -> "abc -> dq (Power-Invariant)"/2(theta), [theta], theta/1
  Saturation/1 -> Sum/1
  Filter p/1 -> Filter p2/1
  Discrete-Time Integrator/1 -> Math Function1/1
  Filter p2/1 -> Discrete PI/2(reference), Scope1/3

== system PLL_fault_experiment/Grid-Following Inverter (Simulink Block)1/PQ Calculation (dq-Frame)1 ==
  note: Power calculation.
      |
      | Author(s): Yitong Li
      |
      | Notes:
      |
      | The calculation is done in dq frame.
  vdq : Inport
  idq : Inport  Port=2
  Mux : Mux  Inputs=2
  Mux1 : Mux  Inputs=2
  P = vd*id+vq*iq : Fcn  Expr=u[1]*u[3]+u[2]*u[4]
  Q = -vd*iq+vq*id : Fcn  Expr=-u[1]*u[4]+u[2]*u[3]
  pq : Outport
  wires:
  Mux/1 -> pq/1
  P = vd*id+vq*iq/1 -> Mux/1
  vdq/1 -> Mux1/1
  idq/1 -> Mux1/2
  Mux1/1 -> P = vd*id+vq*iq/1, Q = -vd*iq+vq*id/1
  Q = -vd*iq+vq*id/1 -> Mux/2

== system PLL_fault_experiment/Grid-Following Inverter (Simulink Block)1/abc -> dq (Power-Invariant)1 ==
  note: Frame transformation from abc to dq.
      |
      | Author(s): Yitong Li
      |
      | Notes:
      |
      | The transformation is power-invariant.
      |
      | theta is the angle that d axis leads a axis.
      |
      | q axis leads d axis by 90 degrees.
  abc : Inport  SampleTime=Tc
  theta : Inport  Port=2  SampleTime=Tc
  ->d : Fcn  Expr=cos(u(4))*u(1) + cos(u(4)-2/3*pi)*u(2) + cos(u(4)-4/3*pi)*u(3)
  ->q : Fcn  Expr=-sin(u(4))*u(1) - sin(u(4)-2/3*pi)*u(2) - sin(u(4)-4/3*pi)*u(3)
  Gain : Gain  Gain=sqrt(2/3)
  Mux5 : Mux  Inputs=2
  Mux6 : Mux  Inputs=2
  dq : Outport  SampleTime=Tc
  wires:
  abc/1 -> Gain/1
  ->d/1 -> Mux6/1
  Gain/1 -> Mux5/1
  theta/1 -> Mux5/2
  ->q/1 -> Mux6/2
  Mux6/1 -> dq/1
  Mux5/1 -> ->d/1, ->q/1

== system PLL_fault_experiment/Grid-Following Inverter (Simulink Block)1/abc -> dq (Power-Invariant)2 ==
  note: Frame transformation from abc to dq.
      |
      | Author(s): Yitong Li
      |
      | Notes:
      |
      | The transformation is power-invariant.
      |
      | theta is the angle that d axis leads a axis.
      |
      | q axis leads d axis by 90 degrees.
  abc : Inport  SampleTime=Tc
  theta : Inport  Port=2  SampleTime=Tc
  ->d : Fcn  Expr=cos(u(4))*u(1) + cos(u(4)-2/3*pi)*u(2) + cos(u(4)-4/3*pi)*u(3)
  ->q : Fcn  Expr=-sin(u(4))*u(1) - sin(u(4)-2/3*pi)*u(2) - sin(u(4)-4/3*pi)*u(3)
  Gain : Gain  Gain=sqrt(2/3)
  Mux5 : Mux  Inputs=2
  Mux6 : Mux  Inputs=2
  dq : Outport  SampleTime=Tc
  wires:
  abc/1 -> Gain/1
  ->d/1 -> Mux6/1
  Gain/1 -> Mux5/1
  theta/1 -> Mux5/2
  ->q/1 -> Mux6/2
  Mux6/1 -> dq/1
  Mux5/1 -> ->d/1, ->q/1

== system PLL_fault_experiment/Grid-Following Inverter (Simulink Block)1/abc -> dq (Power-Invariant)3 ==
  note: Frame transformation from abc to dq.
      |
      | Author(s): Yitong Li
      |
      | Notes:
      |
      | The transformation is power-invariant.
      |
      | theta is the angle that d axis leads a axis.
      |
      | q axis leads d axis by 90 degrees.
  abc : Inport  SampleTime=Tc
  theta : Inport  Port=2  SampleTime=Tc
  ->d : Fcn  Expr=cos(u(4))*u(1) + cos(u(4)-2/3*pi)*u(2) + cos(u(4)-4/3*pi)*u(3)
  ->q : Fcn  Expr=-sin(u(4))*u(1) - sin(u(4)-2/3*pi)*u(2) - sin(u(4)-4/3*pi)*u(3)
  Gain : Gain  Gain=sqrt(2/3)
  Mux5 : Mux  Inputs=2
  Mux6 : Mux  Inputs=2
  dq : Outport  SampleTime=Tc
  wires:
  abc/1 -> Gain/1
  ->d/1 -> Mux6/1
  Gain/1 -> Mux5/1
  theta/1 -> Mux5/2
  ->q/1 -> Mux6/2
  Mux6/1 -> dq/1
  Mux5/1 -> ->d/1, ->q/1

== system PLL_fault_experiment/Grid-Following Inverter (Simulink Block)1/abc -> dq (Power-Invariant)4 ==
  note: Frame transformation from abc to dq.
      |
      | Author(s): Yitong Li
      |
      | Notes:
      |
      | The transformation is power-invariant.
      |
      | theta is the angle that d axis leads a axis.
      |
      | q axis leads d axis by 90 degrees.
  abc : Inport
  theta : Inport  Port=2
  ->d : Fcn  Expr=cos(u(4))*u(1) + cos(u(4)-2/3*pi)*u(2) + cos(u(4)-4/3*pi)*u(3)
  ->q : Fcn  Expr=-sin(u(4))*u(1) - sin(u(4)-2/3*pi)*u(2) - sin(u(4)-4/3*pi)*u(3)
  Gain : Gain  Gain=sqrt(2/3)
  Mux5 : Mux  Inputs=2
  Mux6 : Mux  Inputs=2
  dq : Outport
  wires:
  abc/1 -> Gain/1
  ->d/1 -> Mux6/1
  Gain/1 -> Mux5/1
  theta/1 -> Mux5/2
  ->q/1 -> Mux6/2
  Mux6/1 -> dq/1
  Mux5/1 -> ->d/1, ->q/1

== system PLL_fault_experiment/Grid-Following Inverter (Simulink Block)1/abc -> dq (Power-Invariant)5 ==
  note: Frame transformation from abc to dq.
      |
      | Author(s): Yitong Li
      |
      | Notes:
      |
      | The transformation is power-invariant.
      |
      | theta is the angle that d axis leads a axis.
      |
      | q axis leads d axis by 90 degrees.
  abc : Inport  SampleTime=Tc
  theta : Inport  Port=2  SampleTime=Tc
  ->d : Fcn  Expr=cos(u(4))*u(1) + cos(u(4)-2/3*pi)*u(2) + cos(u(4)-4/3*pi)*u(3)
  ->q : Fcn  Expr=-sin(u(4))*u(1) - sin(u(4)-2/3*pi)*u(2) - sin(u(4)-4/3*pi)*u(3)
  Gain : Gain  Gain=sqrt(2/3)
  Mux5 : Mux  Inputs=2
  Mux6 : Mux  Inputs=2
  dq : Outport  SampleTime=Tc
  wires:
  abc/1 -> Gain/1
  ->d/1 -> Mux6/1
  Gain/1 -> Mux5/1
  theta/1 -> Mux5/2
  ->q/1 -> Mux6/2
  Mux6/1 -> dq/1
  Mux5/1 -> ->d/1, ->q/1

== system PLL_fault_experiment/Grid-Following Inverter (Simulink Block)1/dq -> abc (Power-Invariant)1 ==
  note: Frame transformation from dq to abc.
      |
      | Author(s): Yitong Li
      |
      | Notes:
      |
      | The transformation is power-invariant.
      |
      | theta is the angle that dq axis leads alpha/beta axis, specifically, d axis leads alpha axis.
  dq : Inport  SampleTime=Tc
  theta : Inport  Port=2  SampleTime=Tc
  ->a : Fcn  Expr=cos(u(3))*u(1) - sin(u(3))*u(2)
  ->b : Fcn  Expr=cos(u(3)-2/3*pi)*u(1) - sin(u(3)-2/3*pi)*u(2)
  ->c : Fcn  Expr=cos(u(3)-4/3*pi)*u(1) - sin(u(3)-4/3*pi)*u(2)
  Gain : Gain  Gain=sqrt(2/3)
  Mux5 : Mux  Inputs=2
  Mux6 : Mux  Inputs=3
  abc : Outport
  wires:
  ->b/1 -> Mux6/2
  ->a/1 -> Mux6/1
  Gain/1 -> Mux5/1
  dq/1 -> Gain/1
  ->c/1 -> Mux6/3
  Mux6/1 -> abc/1
  Mux5/1 -> ->b/1, ->a/1, ->c/1
  theta/1 -> Mux5/2

== system PLL_fault_experiment/Grid-Following Inverter (Simulink Block)1/inverter1 ==
  G : Inport
  block : Inport  Port=2
  Data Type Conversion1 : DataTypeConversion  OutDataTypeStr=double  SaturateOnIntegerOverflow=off  RndMeth=Floor
  Data Type Conversion2 : DataTypeConversion  OutDataTypeStr=double  SaturateOnIntegerOverflow=off  RndMeth=Floor
  Data Type Conversion3 : DataTypeConversion  OutDataTypeStr=double  SaturateOnIntegerOverflow=off  RndMeth=Floor
  Data Type Conversion4 : DataTypeConversion  OutDataTypeStr=boolean  SaturateOnIntegerOverflow=off  RndMeth=Floor
  Data Type Conversion5 : DataTypeConversion  OutDataTypeStr=boolean  SaturateOnIntegerOverflow=off  RndMeth=Floor
  Data Type Conversion6 : DataTypeConversion  OutDataTypeStr=boolean  SaturateOnIntegerOverflow=off  RndMeth=Floor
  Demux : Demux  Outputs=3
  Half-Bridge Converter : spsHalfBridgeConverterLib/Half-Bridge Converter  ModelType=Switching devices  Ron=1e-6  Rs=1e6 %10  Cs=inf %0.3e-9  Vforward=[0,0]  Ron_Diode=1e-3  Rs_Diode=1e6  Cs_Diode=inf  Vf_Diode=1e-3  Rs_CurrentSource=inf  Ron_ACsource=1e-3
  Half-Bridge Converter1 : spsHalfBridgeConverterLib/Half-Bridge Converter  ModelType=Switching devices  Ron=1e-6  Rs=1e6 %10  Cs=inf %0.3e-9  Vforward=[0,0]  Ron_Diode=1e-3  Rs_Diode=1e6  Cs_Diode=inf  Vf_Diode=1e-3  Rs_CurrentSource=inf  Ron_ACsource=1e-3
  Half-Bridge Converter2 : spsHalfBridgeConverterLib/Half-Bridge Converter  ModelType=Switching devices  Ron=1e-6  Rs=1e6 %10  Cs=inf %0.3e-9  Vforward=[0,0]  Ron_Diode=1e-3  Rs_Diode=1e6  Cs_Diode=inf  Vf_Diode=1e-3  Rs_CurrentSource=inf  Ron_ACsource=1e-3
  Logical Operator : Logic  Operator=NOT  AllPortsSameDT=off  OutDataTypeStr=boolean
  Logical Operator1 : Logic  Operator=NOT  AllPortsSameDT=off  OutDataTypeStr=boolean
  Logical Operator2 : Logic  Operator=NOT  AllPortsSameDT=off  OutDataTypeStr=boolean
  Mux : Mux  Inputs=2
  Mux1 : Mux  Inputs=2
  Mux2 : Mux  Inputs=2
  Scope : Scope
      settings: ActiveDisplayYMinimum=-0.17937  ActiveDisplayYMaximum=2.81832  DataLoggingVariableName=ScopeData4
  Scope1 : Scope
      settings: ActiveDisplayYMinimum=-0.03009  ActiveDisplayYMaximum=1.07279  DataLoggingVariableName=ScopeData5
  Vbc1 : spsVoltageMeasurementLib/Voltage Measurement  PhasorSimulation=off  OutputType=Complex  PSBequivalent=0
  DC+ : PMIOPort  Tag=PMCPort  Side=Left
  DC- : PMIOPort  Tag=PMCPort  Port=2  Side=Left
  A : PMIOPort  Tag=PMCPort  Port=3  Side=Right
  B : PMIOPort  Tag=PMCPort  Port=4  Side=Right
  C : PMIOPort  Tag=PMCPort  Port=5  Side=Right
  wires:
  G/1 -> Demux/1
  block/1 -> Half-Bridge Converter/2, Half-Bridge Converter2/2, Half-Bridge Converter1/2
  Demux/1 -> Data Type Conversion4/1, Mux/1
  Logical Operator/1 -> Data Type Conversion1/1
  Demux/2 -> Mux1/1, Data Type Conversion5/1
  Logical Operator1/1 -> Data Type Conversion2/1
  Demux/3 -> Mux2/1, Data Type Conversion6/1
  Logical Operator2/1 -> Data Type Conversion3/1
  Mux/1 -> Scope1/1, Half-Bridge Converter/1
  Mux1/1 -> Half-Bridge Converter1/1
  Mux2/1 -> Half-Bridge Converter2/1
  Data Type Conversion4/1 -> Logical Operator/1
  Data Type Conversion5/1 -> Logical Operator1/1
  Data Type Conversion6/1 -> Logical Operator2/1
  Data Type Conversion1/1 -> Mux/2
  Data Type Conversion2/1 -> Mux1/2
  Data Type Conversion3/1 -> Mux2/2
  Vbc1/1 -> Scope/1
  connections:
  C/RConn1 -- Half-Bridge Converter2/LConn1
  B/RConn1 -- Half-Bridge Converter1/LConn1
  A/RConn1 -- Vbc1/LConn1 -- Half-Bridge Converter/LConn1
  DC+/RConn1 -- Half-Bridge Converter2/RConn1 -- Half-Bridge Converter1/RConn1 -- Half-Bridge Converter/RConn1
  Half-Bridge Converter/RConn2 -- Vbc1/LConn2 -- Half-Bridge Converter1/RConn2 -- Half-Bridge Converter2/RConn2 -- DC-/RConn1
